simulink model "single_phase_constant_power"  (Simulink 8.1)
settings: Solver=FixedStepDiscrete  StartTime=0.0  StopTime=60  FixedStep=1  MaxStep=1/60  RelTol=1e-3
InitFcn:
  | Ts = 1e-5;
libraries: powerlib x7, simulink x2, CampusEnergyModeling x1, powerlib_meascontrol x1
settings Model: Creator=sfrank1  LastModifiedBy=sfrank1

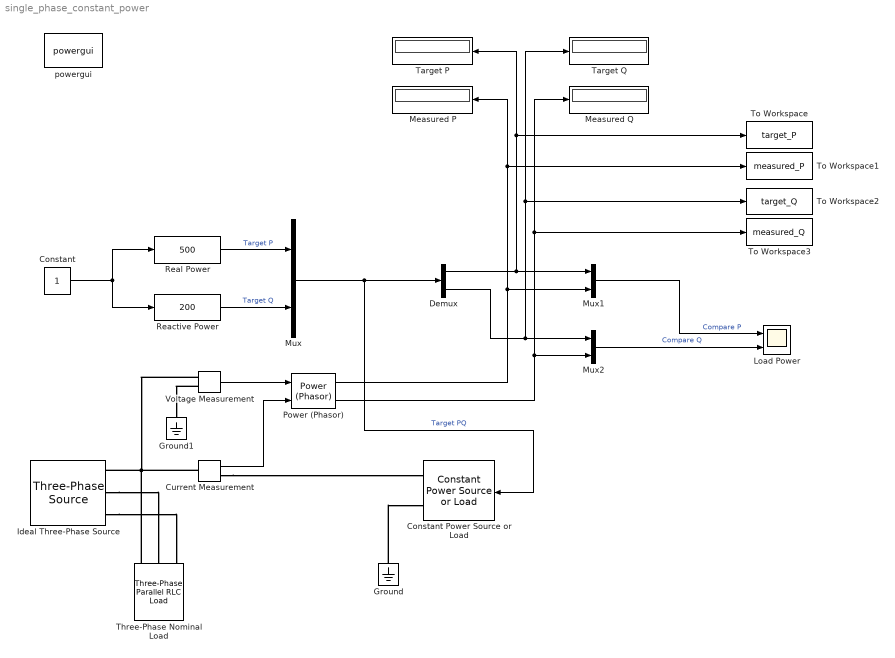
== system single_phase_constant_power ==
  Constant : Constant
  Constant Power Source or Load : CampusEnergyModeling/Electrical/Constant Power Source or Load  Conven=load  PNom=1000  QNom=0  VNom=120  fNom=60  VLow=0.7
  Current Measurement : powerlib/Measurements/Current Measurement  PhasorSimulation=on  OutputType=Complex  PSBequivalent=0
  Demux : Demux  Outputs=2
  Ground : powerlib/Elements/Ground  LConnTagsString=a
  Ground1 : powerlib/Elements/Ground  LConnTagsString=a
  Ideal Three-Phase Source : powerlib/Electrical Sources/Three-Phase Source  Voltage=208  PhaseAngle=0  Frequency=60  InternalConnection=Yg  SpecifyImpedance=on  Resistance=0  Inductance=0  ShortCircuitLevel=1e6  BaseVoltage=208  XRratio=1  BusType=swing  Pref=0  Qref=0  Qmin=-inf  Qmax=inf
  Load Power : Scope  NumInputPorts=2
      settings: TickLabels=on  TimeRange=60  YMin=400~0  YMax=1000~250
  Measured P : Display
  Measured Q : Display
  Mux : Mux  Inputs=2
  Mux1 : Mux  Inputs=2
  Mux2 : Mux  Inputs=2
  Power (Phasor) : powerlib_meascontrol/Measurements/Power (Phasor)
  Reactive Power : simulink/Math Operations/Slider Gain  low=-1000  gain=200  high=1000
  Real Power : simulink/Math Operations/Slider Gain  low=-1000  gain=500  high=1000
  Target P : Display
  Target Q : Display
  Three-Phase Nominal Load : powerlib/Elements/Three-Phase Parallel RLC Load  LConnTagsString=A|B|C  Configuration=Delta  NominalVoltage=208  NominalFrequency=60  ActivePower=1  InductivePower=0  CapacitivePower=0  Measurements=None  LoadType=constant Z
  To Workspace : ToWorkspace  VariableName=target_P  SampleTime=-1
      settings: MaxDataPoints=1
  To Workspace1 : ToWorkspace  VariableName=measured_P  SampleTime=-1
      settings: MaxDataPoints=1
  To Workspace2 : ToWorkspace  VariableName=target_Q  SampleTime=-1
      settings: MaxDataPoints=1
  To Workspace3 : ToWorkspace  VariableName=measured_Q  SampleTime=-1
      settings: MaxDataPoints=1
  Voltage Measurement : powerlib/Measurements/Voltage Measurement  PhasorSimulation=on  OutputType=Complex  PSBequivalent=0
  powergui : powerlib/powergui  Priority=1  SimulationMode=Phasor  SolverType=Tustin  SampleTime=50e-6  frequency=60  SPID=off  DisableSnubberDevices=off  DisableRonSwitches=off  DisableVfSwitches=off  SwTol=0  Interpol=off  DisplayEquations=off  frequencyindice=60  Pbase=100e3  ErrMax=1e-4  Iterations=50  UnitsV=kV  UnitsW=MW  FunctionMessages=off  echomessages=off  HookPort=off  EnableUseOfTLC=off  x0status=blocks  RestoreLinks=warning  ResistiveCurrentMeasurement=off  Frange=[0:2:500]  Ylog=off  Xlog=on  ShowGrid=off  save=off  variable=ZData  ZoomFFT=off  StartTime=0.0  cycles=1  DisplayStyle=1  fundamental=60  FreqAxis=off  MaxFrequency=1000  frequencyindicesteady=1  RmsSteady=1  display=off  Ts=0  methode=off
  wires:
  Constant/1 -> Reactive Power/1, Real Power/1
  Real Power/1 -> Mux/1  "Target P"
  Mux/1 -> Constant Power Source or Load/1, Demux/1  "Target PQ"
  Reactive Power/1 -> Mux/2  "Target Q"
  Mux1/1 -> Load Power/1  "Compare P"
  Mux2/1 -> Load Power/2  "Compare Q"
  Demux/1 -> Mux1/1, To Workspace/1, Target P/1
  Power (Phasor)/1 -> To Workspace1/1, Measured P/1, Mux1/2
  Demux/2 -> Mux2/1, To Workspace2/1, Target Q/1
  Power (Phasor)/2 -> Mux2/2, To Workspace3/1, Measured Q/1
  Current Measurement/1 -> Power (Phasor)/2
  Voltage Measurement/1 -> Power (Phasor)/1
  connections:
  Three-Phase Nominal Load/LConn1 -- Voltage Measurement/LConn1 -- Current Measurement/LConn1 -- Ideal Three-Phase Source/RConn1
  Ground/LConn1 -- Constant Power Source or Load/RConn2
  Ideal Three-Phase Source/RConn2 -- Three-Phase Nominal Load/LConn2
  Ideal Three-Phase Source/RConn3 -- Three-Phase Nominal Load/LConn3
  Current Measurement/RConn1 -- Constant Power Source or Load/RConn1
  Voltage Measurement/LConn2 -- Ground1/LConn1
